simulink model "joint_control_system"  (R2015a)
settings: Solver=FixedStepDiscrete  StartTime=0.0  StopTime=10  FixedStep=0.02  RelTol=1e-3
values from neighbouring files (symbols this model uses):
  A = stateModelMatrices(1:l-1, 1:l-1)    [controller_design_1.m]    (also in controller_design_2.m)
  B = stateModelMatrices(1:l-1, l)    [controller_design_1.m]    (also in controller_design_2.m)
  C = stateModelMatrices(l, 1:l-1)    [controller_design_1.m]    (also in controller_design_2.m)
  D = stateModelMatrices(l, l)    [controller_design_1.m]    (also in controller_design_2.m)
  Nbar = Nu+K*Nx    [controller_design_1.m]    (also in controller_design_2.m)
undefined symbols (not defined in the file or in its folder): K, M
settings Model: CovModelRefEnable=off  Creator=João  LastModifiedBy=luisr
settings DataIOCC: SaveFormat=Dataset
settings HardwareCC: ProdBitPerPointer=64  ProdLargestAtomicFloat=Float  ProdIntDivRoundTo=Zero  ProdEndianess=LittleEndian  ProdHWDeviceType=Specified
settings GRTTargetCC: GeneratePreprocessorConditionals=Use local settings

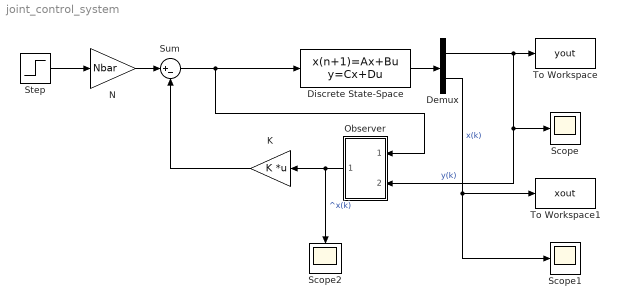
== system joint_control_system ==
  Demux : Demux  Outputs=[1 4]
  Discrete State-Space : DiscreteStateSpace  A=A  B=B  C=[C; eye(length(A))]  D=[D; zeros(size(A,1),1)]  SampleTime=0.02
  K : Gain  Gain=K  Multiplication=Matrix(K*u)
  N : Gain  Gain=Nbar
  Observer : Subsystem
  Scope : Scope
      settings: TimeRange=auto  MaxDataPoints=5000  SaveToWorkspace=off  SaveName=ScopeData  YMin=-1.32807  YMax=1.32791  SampleTime=-1
  Scope1 : Scope
      settings: TimeRange=auto  MaxDataPoints=5000  SaveToWorkspace=off  YMin=-1.32807  YMax=1.32791  SampleTime=-1
  Scope2 : Scope
      settings: TimeRange=auto  MaxDataPoints=5000  SaveToWorkspace=off  SaveName=ScopeData2  YMin=-1.32807  YMax=1.32791  SampleTime=-1
  Step : Step  Time=5  SampleTime=0
  Sum : Sum  Inputs=|+-
  To Workspace : ToWorkspace  VariableName=yout  SaveFormat=Structure With Time  SampleTime=-1
  To Workspace1 : ToWorkspace  VariableName=xout  SaveFormat=Structure With Time  SampleTime=-1
  wires:
  Step/1 -> N/1
  N/1 -> Sum/1
  Sum/1 -> Observer/1(In1), Discrete State-Space/1
  K/1 -> Sum/2
  Observer/1(Out1) -> K/1, Scope2/1  "^x(k)"
  Discrete State-Space/1 -> Demux/1
  Demux/1 -> Observer/2(In2), Scope/1, To Workspace/1  "y(k)"
  Demux/2 -> Scope1/1, To Workspace1/1  "x(k)"

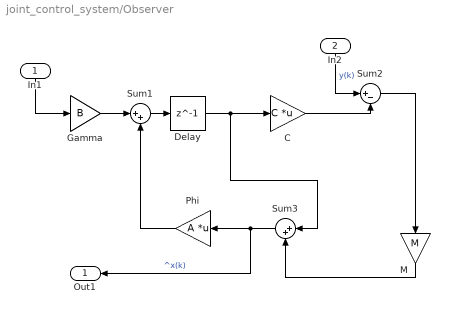
== system joint_control_system/Observer ==
  In1 : Inport
  In2 : Inport  Port=2
  C : Gain  Gain=C  Multiplication=Matrix(K*u)
  Delay : Delay  DelayLength=1  InitialCondition=0  SampleTime=[0.02,0]
  Gamma : Gain  Gain=B
  M : Gain  Gain=M
  Phi : Gain  Gain=A  Multiplication=Matrix(K*u)
  Sum1 : Sum  Inputs=|++
  Sum2 : Sum  Inputs=|+-
  Sum3 : Sum  Inputs=|++
  Out1 : Outport
  wires:
  In1/1 -> Gamma/1
  In2/1 -> Sum2/1  "y(k)"
  Gamma/1 -> Sum1/1
  Sum1/1 -> Delay/1
  Delay/1 -> Sum3/1, C/1
  Sum2/1 -> M/1
  C/1 -> Sum2/2
  Phi/1 -> Sum1/2
  Sum3/1 -> Out1/1, Phi/1  "^x(k)"
  M/1 -> Sum3/2
